simulink model "Cau_3_1011"  (R2016b)
settings: Solver=ode4  StartTime=0.0  StopTime=1  FixedStep=1e-4  RelTol=1e-3
settings Model: Creator=ADMIN  LastModifiedBy=ADMIN

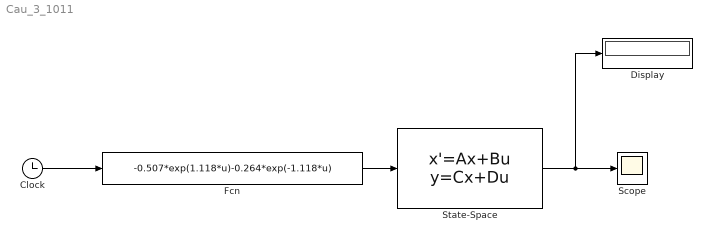
== system Cau_3_1011 ==
  Clock : Clock
  Display : Display
  Fcn : Fcn  Expr=-0.507*exp(1.118*u)-0.264*exp(-1.118*u)
  Scope : Scope
  State-Space : StateSpace  A=-1  B=0.5  D=0  X0=1
  wires:
  Clock/1 -> Fcn/1
  Fcn/1 -> State-Space/1
  State-Space/1 -> Display/1, Scope/1
